simulink model "quick_test"  (R2019a)
settings: Solver=ode14x  StartTime=0.0  StopTime=1.5  FixedStep=1e-5  RelTol=1e-3
libraries: dsparch4 x3
settings Model: Creator=marco  LastModifiedBy=marco
settings DebuggingCC: SigSpecEnsureSampleTimeMsg=none

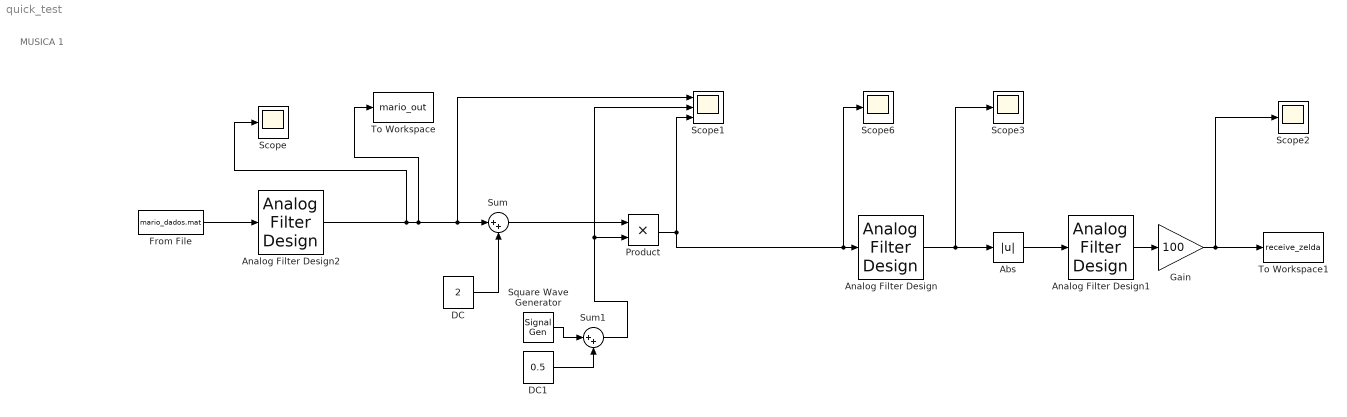
== system quick_test ==
  note: MUSICA 1
  Abs : Abs
  Analog Filter Design : dsparch4/Analog Filter Design  method=Butterworth  filttype=Bandpass  N=5  Wlo=2*pi*102e3  Whi=2*pi*108e3  Rp=2  Rs=40
  Analog Filter Design1 : dsparch4/Analog Filter Design  method=Butterworth  filttype=Lowpass  N=5  Wlo=2*pi*30e3  Whi=2*pi*1020e3  Rp=2  Rs=40
  Analog Filter Design2 : dsparch4/Analog Filter Design  method=Butterworth  filttype=Lowpass  N=10  Wlo=2*pi*5e3  Whi=2*pi*1020e3  Rp=2  Rs=40
  DC : Constant  Value=2
  DC1 : Constant  Value=0.5
  From File : FromFile  FileName=mario_dados.mat  SampleTime=0  ExtrapolationBeforeFirstDataPoint=Ground value
  Gain : Gain  Gain=100
  Product : Product
  Scope{,2..3,6} (4 alike) : Scope
  Scope1 : Scope  NumInputPorts=3
  Square Wave Generator : SignalGenerator  WaveForm=square  Amplitude=0.5  Frequency=105e3
  Sum : Sum  Inputs=|++
  Sum1 : Sum  Inputs=|++
  To Workspace : ToWorkspace  VariableName=mario_out  SaveFormat=Timeseries  SampleTime=1e-5
  To Workspace1 : ToWorkspace  VariableName=receive_zelda  SaveFormat=Timeseries  SampleTime=1e-5
  wires:
  Sum/1 -> Product/1
  DC/1 -> Sum/2
  Sum1/1 -> Scope1/2, Product/2
  Analog Filter Design/1 -> Scope3/1, Abs/1
  Abs/1 -> Analog Filter Design1/1
  From File/1 -> Analog Filter Design2/1
  Analog Filter Design2/1 -> Scope1/1, Sum/1, To Workspace/1, Scope/1
  Square Wave Generator/1 -> Sum1/1
  DC1/1 -> Sum1/2
  Product/1 -> Analog Filter Design/1, Scope6/1, Scope1/3
  Analog Filter Design1/1 -> Gain/1
  Gain/1 -> Scope2/1, To Workspace1/1
